simulink model "problem3"  (R2024b)
settings: Solver=VariableStepAuto  StartTime=0.0  StopTime=100  RelTol=1e-3
model workspace (MAT data in the model file):
  a_m = 0.7408
  b_m = 0.2592
settings Model: Creator=djd14  LastModifiedBy=djd14

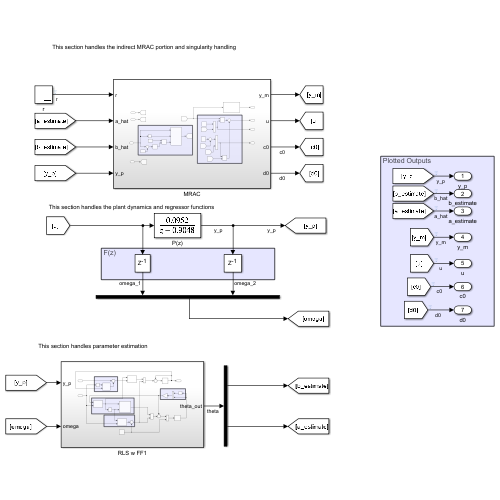
[thumbnail: Simulink's stored preview of the top-level diagram]
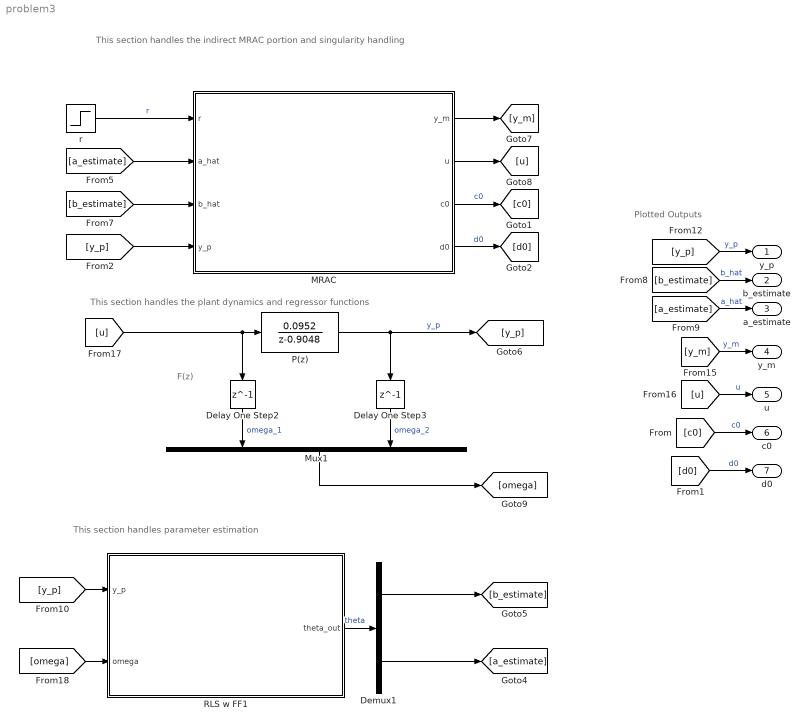
== system problem3 ==
  note: This section handles the indirect MRAC portion and singularity handling
  note: This section handles the plant dynamics and regressor functions
  note: F(z)
  note: Plotted Outputs
  note: This section handles parameter estimation
  Delay One Step2 : Delay  DelayLength=1
  Delay One Step3 : Delay  DelayLength=1
  Demux1 : Demux  Outputs=2
  MRAC : Subsystem
  Mux1 : Mux  Inputs=2
  P(z) : DiscreteTransferFcn  Numerator=[0.0952]  Denominator=[1 -0.9048]
  RLS w FF1 : Subsystem
  r : Step  Time=50  Before=1  After=-1  SampleTime=0
  y_p : Outport  SampleTime=1
  b_estimate : Outport  Port=2
  a_estimate : Outport  Port=3
  y_m : Outport  Port=4
  u : Outport  Port=5
  c0 : Outport  Port=6
  d0 : Outport  Port=7
  wires:
  [y_p] -> y_p/1  "y_p"
  [a_estimate] -> a_estimate/1  "a_hat"
  Delay One Step3/1 -> Mux1/2  "omega_2"
  [u] -> P(z)/1, Delay One Step2/1
  [y_p] -> RLS w FF1/1(y_p)
  [u] -> u/1  "u"
  [y_m] -> y_m/1  "y_m"
  P(z)/1 -> [y_p], Delay One Step3/1  "y_p"
  [omega] -> RLS w FF1/2(omega)
  RLS w FF1/1(theta_out) -> Demux1/1  "theta"
  Demux1/2 -> [a_estimate]
  Mux1/1 -> [omega]
  [b_estimate] -> b_estimate/1  "b_hat"
  Demux1/1 -> [b_estimate]
  Delay One Step2/1 -> Mux1/1  "omega_1"
  r/1 -> MRAC/1(r)  "r"
  [a_estimate] -> MRAC/2(a_hat)
  [b_estimate] -> MRAC/3(b_hat)
  [y_p] -> MRAC/4(y_p)
  MRAC/1(y_m) -> [y_m]
  MRAC/2(u) -> [u]
  MRAC/3(c0) -> [c0]  "c0"
  MRAC/4(d0) -> [d0]  "d0"
  [c0] -> c0/1  "c0"
  [d0] -> d0/1  "d0"

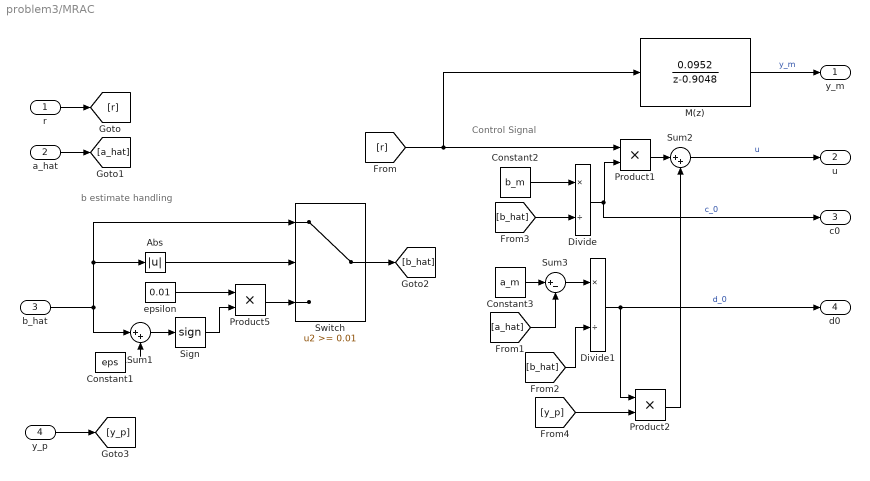
== system problem3/MRAC ==
  note: Control Signal
  note: b estimate handling
  r : Inport
  a_hat : Inport  Port=2
  b_hat : Inport  Port=3
  y_p : Inport  Port=4
  Abs : Abs  SaturateOnIntegerOverflow=off
  Constant1 : Constant  Value=eps
  Constant2 : Constant  Value=b_m
  Constant3 : Constant  Value=a_m
  Divide : Product  Inputs=*/
  Divide1 : Product  Inputs=*/
  M(z) : DiscreteTransferFcn  Numerator=[0.0952]  Denominator=[1 -0.9048]
  Product1 : Product
  Product2 : Product
  Product5 : Product
  Sign : Signum  ZeroCross=off
  Sum1 : Sum  Inputs=|++
  Sum2 : Sum  Inputs=|++
  Sum3 : Sum  Inputs=|+-
  Switch : Switch  Threshold=0.01  SaturateOnIntegerOverflow=off  InputSameDT=off
  epsilon : Constant  Value=0.01
  y_m : Outport
  u : Outport  Port=2
  c0 : Outport  Port=3
  d0 : Outport  Port=4
  wires:
  [b_hat] -> Divide/2
  Product2/1 -> Sum2/2
  Sum3/1 -> Divide1/1
  Constant3/1 -> Sum3/1
  Product1/1 -> Sum2/1
  Divide1/1 -> d0/1, Product2/1  "d_0"
  [y_p] -> Product2/2
  Constant2/1 -> Divide/1
  [r] -> M(z)/1, Product1/1
  Divide/1 -> c0/1, Product1/2  "c_0"
  Sum2/1 -> u/1  "u"
  M(z)/1 -> y_m/1  "y_m"
  [b_hat] -> Divide1/2
  [a_hat] -> Sum3/2
  r/1 -> [r]
  a_hat/1 -> [a_hat]
  y_p/1 -> [y_p]
  Abs/1 -> Switch/2
  epsilon/1 -> Product5/1
  Product5/1 -> Switch/3
  Sign/1 -> Product5/2
  Switch/1 -> [b_hat]
  b_hat/1 -> Sum1/1, Switch/1, Abs/1
  Sum1/1 -> Sign/1
  Constant1/1 -> Sum1/2

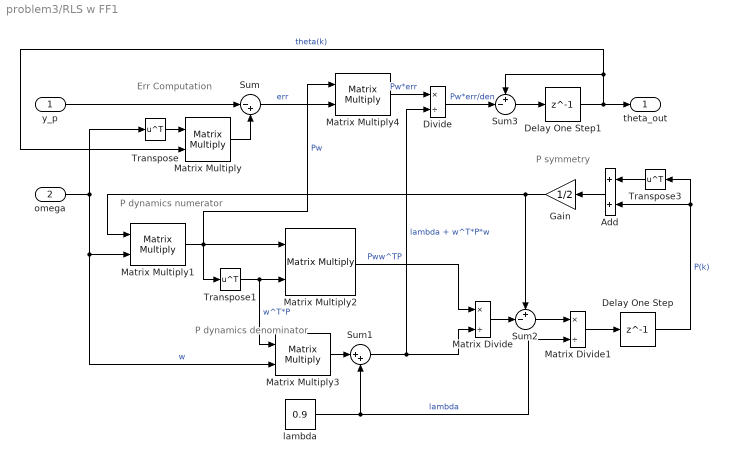
== system problem3/RLS w FF1 ==
  note: P symmetry
  note: P dynamics denominator
  note: P dynamics numerator
  note: Err Computation
  y_p : Inport
  omega : Inport  Port=2
  Add : Sum
  Delay One Step : Delay  DelayLength=1  InitialCondition=100*eye(2)
  Delay One Step1 : Delay  DelayLength=1  InitialCondition=[0 0]
  Divide : Product  Inputs=*/
  Gain : Gain  Gain=1/2
  Matrix Divide : Product  Inputs=*/
  Matrix Divide1 : Product  Inputs=*/
  Matrix Multiply{,1..4} (5 alike) : Product  Multiplication=Matrix(*)
  Sum : Sum  Inputs=|-+
  Sum1 : Sum  Inputs=|++
  Sum2 : Sum  Inputs=+-|
  Sum3 : Sum  Inputs=+-|
  Transpose : Math  Operator=transpose
  Transpose1 : Math  Operator=transpose
  Transpose3 : Math  Operator=transpose
  lambda : Constant  Value=0.9
  theta_out : Outport
  wires:
  omega/1 -> Transpose/1, Matrix Multiply3/2, Matrix Multiply1/2  "w"
  Transpose/1 -> Matrix Multiply/1
  y_p/1 -> Sum/1
  Matrix Multiply/1 -> Sum/2
  Sum/1 -> Matrix Multiply4/2  "err"
  Matrix Multiply1/1 -> Matrix Multiply4/1, Matrix Multiply2/1, Transpose1/1  "Pw"
  Delay One Step/1 -> Transpose3/1, Add/2  "P(k)"
  Matrix Multiply2/1 -> Matrix Divide/1  "Pww^TP"
  Transpose1/1 -> Matrix Multiply3/1, Matrix Multiply2/2  "w^T*P"
  Matrix Multiply3/1 -> Sum1/1
  Sum1/1 -> Divide/2, Matrix Divide/2  "lambda + w^T*P*w"
  Matrix Divide/1 -> Sum2/2
  Sum2/1 -> Matrix Divide1/1
  Matrix Divide1/1 -> Delay One Step/1
  Transpose3/1 -> Add/1
  Add/1 -> Gain/1
  Gain/1 -> Matrix Multiply1/1, Sum2/1
  lambda/1 -> Matrix Divide1/2, Sum1/2  "lambda"
  Sum3/1 -> Delay One Step1/1
  Delay One Step1/1 -> theta_out/1, Matrix Multiply/2, Sum3/1  "theta(k)"
  Matrix Multiply4/1 -> Divide/1  "Pw*err"
  Divide/1 -> Sum3/2  "Pw*err/den"
